simulink model "Simulation_balancenew2024versionajour"  (R2024a)
settings: Solver=ode4  StartTime=0.0  StopTime=1  FixedStep=step_time  RelTol=1e-3
InitFcn:
  | Initialisation_simulation
values from neighbouring files (symbols this model uses):
  denom_com = [R^2*C^2 3*R*C 1]    [Initialisation_simulation.m]
  denom_cou = [1/(2*pi*165) 1]    [Initialisation_simulation.m]
  denom_pos = [1/(2*pi*80) 1]    [Initialisation_simulation.m]
  denom_proc = [1,551.329784176462,25092.4669239778,5556154.83244325,117762820.943339,13657291814.2789,114001597319.831]    [Initialisation_simulation.m]
  dL_table = LUT_Table{:,6}    [Initialisation_simulation.m]
  dPhi_table = LUT_Table{:,7}    [Initialisation_simulation.m]
  gain_com = 0.88    [Initialisation_simulation.m]
  gain_cou = 0.716    [Initialisation_simulation.m]
  gain_mod_cou = Gain_Ampli_Puissance(1)    [Initialisation_simulation.m]
  gain_pos = 1.4925    [Initialisation_simulation.m]
  gain_puis = Gain_Ampli_Puissance(1)    [Initialisation_simulation.m]
  kb_table = LUT_Table{:,5}    [Initialisation_simulation.m]
  ki_courant = -325    [Initialisation_simulation.m]
  kp_courant = -0.575    [Initialisation_simulation.m]
  Lb_table = LUT_Table{:,4}    [Initialisation_simulation.m]
  num_com = 1    [Initialisation_simulation.m]
  num_cou = 1    [Initialisation_simulation.m]
  num_pos = 1    [Initialisation_simulation.m]
  num_proc = [0,0,0,-2365575.26407082,-23596424.4747652,-9504262175.32001,-113750992077.689]    [Initialisation_simulation.m]
  offset_com = -2.5    [Initialisation_simulation.m]
  offset_cou = 3.44    [Initialisation_simulation.m]
  offset_pos = -1.6    [Initialisation_simulation.m]
  per_adc = 1/freq_adc    (= 0.000166666666667)    [Initialisation_simulation.m]
  per_pwm = 1/freq_pwm    (= 6.4e-05)    [Initialisation_simulation.m]
  rb = 1.1745 + 2.349    (= 3.5235)    [Initialisation_simulation.m]
  ref_pos_act = 10    [Initialisation_simulation.m]
  ref_pos_proc = 8e-3    (= 0.008)    [Initialisation_simulation.m]
  sat_com_max = 5    [Initialisation_simulation.m]
  sat_com_min = -5    [Initialisation_simulation.m]
  sat_cou_max = 5    [Initialisation_simulation.m]
  sat_cou_min = 0    [Initialisation_simulation.m]
  sat_pos_max = 5    [Initialisation_simulation.m]
  sat_pos_min = 0    [Initialisation_simulation.m]
  sat_proc_max = 14e-3    (= 0.014)    [Initialisation_simulation.m]    (also in beam_build_ss.m = 1; lookup_table_statespace.m = 1)
  sat_proc_min = 0    [Initialisation_simulation.m]    (also in beam_build_ss.m = -1; lookup_table_statespace.m = -1)
  sat_puis_max = 5    [Initialisation_simulation.m]
  sat_puis_min = -5    [Initialisation_simulation.m]
  step_time = 1/300000    (= 3.33333333333e-06)    [Initialisation_simulation.m]
  tension_selon_distance = polyfit(Distance(1:point_final), Tension(1:point_final), 3)    [Initialisation_simulation.m]
  x_table = LUT_Table{:,2}    [Initialisation_simulation.m]
libraries: simulink_extras x2, slpidlib x2, simulink x2
settings Model: DataTypeOverride=Double  MinMaxOverflowLogging=ForceOff  Creator=johen30  LastModifiedBy=etmal6

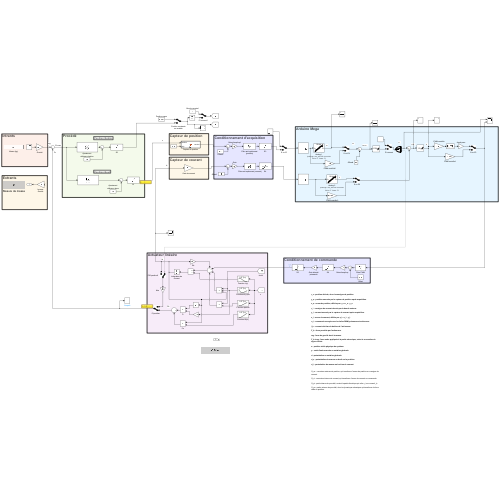
[thumbnail: Simulink's stored preview of the top-level diagram]
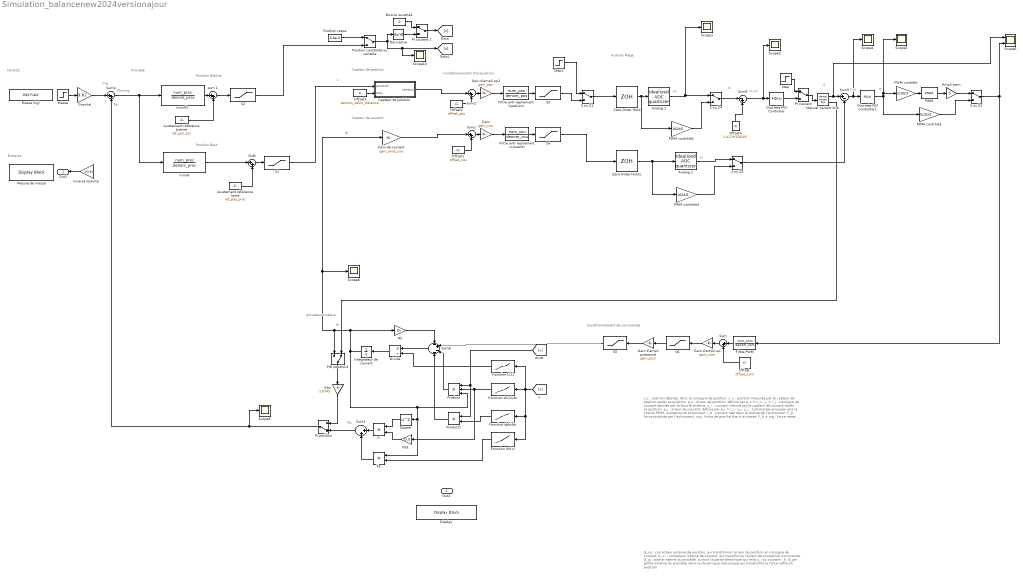
== system Simulation_balancenew2024versionajour ==
  note: G_ce : correcteur externe de position, qui transforme l’erreur de position en consigne de courant.
      |
      | G_ci : correcteur interne de courant, qui transforme l’erreur de courant en commande.
      |
      | G_pi : partie interne du procédé, surtout la partie électrique qui relie u_i au courant i_b.
      |
      | G_pe : partie externe du procédé, donc la dynamique mécanique qui transforme la force nette en position.
  note: r_x : position désirée, donc la consigne de position.
      |
      | y_x : position mesurée par le capteur de position après acquisition.
      |
      | e_x : erreur de position, définie par e_x = r_x - y_x.
      |
      | r_i : consigne de courant donnée par la boucle externe.
      |
      | y_i : courant mesuré par le capteur de courant après acquisition.
      |
      | e_i : erreur de courant, définie par e_i = r_i - y_i.
      |
      | u_i : commande envoyée vers la chaîne PWM, puissance et actionneur.
      |
      | i_b : courant réel dans la bobine de l’actionneur.
      |
      | F_b : force produite par l’actionneur.
      |
      | mg : force de gravité due à la masse.
      |
      | F_b ± mg : force nette appliquée à la partie mécanique, selon la convention de signe choisie.
      |
      | x : position réelle physique du système.
      |
      | y : sortie finale mesurée en notation générale.
      |
      | d : perturbation en notation générale.
      |
      | d_x : perturbation de mesure ou bruit sur la position.
      |
      | d_i : perturbation de mesure ou bruit sur le courant.
  note: Fb
  note: Position Bobine
  note: Extrants
  note: Intrants
  note: Arduino Mega
  note: Procédé
  note: Conditionnement de commande
  note: Conditionnement d'acquisition
  note: Actuateur linéaire
  note: Capteur de courant
  note: Capteur de position
  note: Position Bout
  note: Fb
  note: mg
  note: Fb+mg
  note: x
  note: ib
  note: ib
  note: yx
  note: yi
  note: rx
  note: ri
  note: ri-yi
  note: rx-yx
  note: ui
  Ajustement référence bobine : Constant  Value=ref_pos_act
  Ajustement référence lame : Constant  Value=ref_pos_proc
  Ampli pwm : Gain  Gain=5
  Analog 1 : simulink_extras/Additional Discrete/Idealized ADC quantizer  NumberOfConverterBits=res_adc  Vmin=0  Vmax=5  OutputDataType=int16  OutputNegativeValues=off
  Analog 2 : simulink_extras/Additional Discrete/Idealized ADC quantizer  NumberOfConverterBits=res_adc  Vmin=0  Vmax=5  OutputDataType=int16  OutputNegativeValues=off
  Boucle ouverte1 : Constant  Value=0
  Capteur de position : MATLAB Function  TreatAsAtomicUnit=on
  Derivative : Derivative
  Discrete PID Controller : slpidlib/PID Controller  Controller=PID  Form=Parallel  TimeDomain=Discrete-time  UseExternalTs=off  SampleTime=1/600  IntegratorMethod=Forward Euler  FilterMethod=Forward Euler  ControllerParametersSource=internal  P=-3.75782268839359e-06 * 200  I=-6.64373738618621e-05 * 200  UseKiTs=off  D=4.86414989946578e-07 * 200  UseExternalDerivativeSource=off  N=7.54358045778782  UseFilter=on  TunerSelectOption=Transfer Function Based (PID Tuner App)  InitialConditionSource=internal  InitialConditionForIntegrator=0  InitialConditionForFilter=0  DifferentiatorICPrevScaledInput=0  ExternalReset=none  TrackingMode=off  Kt=1  LimitOutput=on  SatLimitsSource=internal  UpperSaturationLimit=593.34  LowerSaturationLimit=0  LinearizeAsGain=off  AntiWindupMode=none  Kb=1  LimitIntegrator=off  UpperIntegratorSaturationLimit=inf  LowerIntegratorSaturationLimit=-inf  POutMin=[]  POutMax=[]  IOutMin=[]  IOutMax=[]  DOutMin=[]  DOutMax=[]  NOutMin=[]  NOutMax=[]  SumOutMin=[]  SumOutMax=[]  SaturationOutMin=[]  SaturationOutMax=[]  PParamMin=[]  PParamMax=[]  IParamMin=[]  IParamMax=[]  DParamMin=[]  DParamMax=[]  NParamMin=[]  NParamMax=[]  KbParamMin=[]  KbParamMax=[]  KtParamMin=[]  KtParamMax=[]  KbOutMin=[]  KbOutMax=[]  KtOutMin=[]  KtOutMax=[]  IntegratorOutMin=[]  IntegratorOutMax=[]  FilterOutMin=[]  FilterOutMax=[]  SumI1OutMin=[]  SumI1OutMax=[]  SumI2OutMin=[]  SumI2OutMax=[]  SumI3OutMin=[]  SumI3OutMax=[]  SumI4OutMin=[]  SumI4OutMax=[]  SumDOutMin=[]  SumDOutMax=[]  DifferentiatorOutMin=[]  DifferentiatorOutMax=[]  FilterDiffOutCoefMin=[]  FilterDiffOutCoefMax=[]  ReciprocalOutMin=[]  ReciprocalOutMax=[]  SumDenOutMin=[]  SumDenOutMax=[]  SumNumOutMin=[]  SumNumOutMax=[]  DivideOutMin=[]  DivideOutMax=[]  UdiffTsProdOutMin=[]  UdiffTsProdOutMax=[]  NTsProdOutMin=[]  NTsProdOutMax=[]  UintegralTsProdOutMin=[]  UintegralTsProdOutMax=[]  UngainTsProdOutMin=[]  UngainTsProdOutMax=[]  ClampingZeroOutDataTypeStr=Inherit: Inherit via back propagation  ClampingZeroOutMin=[]  ClampingZeroOutMax=[]  FilterDenConstantOutDataTypeStr=Inherit: Inherit via back propagation  FilterDenConstantOutMin=[]  FilterDenConstantOutMax=[]  PCopyOutDataTypeStr=Inherit: Inherit via back propagation  PCopyOutMin=[]  PCopyOutMax=[]  NCopyOutDataTypeStr=Inherit: Inherit via back propagation  NCopyOutMin=[]  NCopyOutMax=[]  IntegratorContinuousStateAttributes=''  IntegratorStateMustResolveToSignalObject=off  IntegratorRTWStateStorageClass=Auto  FilterContinuousStateAttributes=''  FilterStateMustResolveToSignalObject=off  FilterRTWStateStorageClass=Auto  ParallelPVariant=InternalParameters  IdealPVariant=Disabled  IVariant=InternalParameters  DVariant=InternalParameters  IntegratorVariant=Discrete  SatVariant=Enabled  AWVariant=Passthrough  PCopyVariant=Disabled  TRVariant=Disabled  FdbkBlocksVariant=Forward  IdealPFdbkVariant=Disabled  SatFdbkVariant=Disabled  DerivativeFilterVariant=ForwardEulerFilter  NVariant=InternalParameters  NCopyVariant=Disabled  FilterICVariant=InternalICsFilter  IntegratorICVariant=InternalICs  ExternalResetVariant=Disabled  TRSumVariant=Passthrough  SumFdbkVariant=Disabled  SumVariant=Sum_PID  TsampFilterVariant=InternalTs  TsampNgainVariant=Passthrough  TsampIntegralVariant=Disabled_SignalSpec  ExternalSaturationOutDataTypeStr=Inherit: Same as second input  DerivativeSourceVariant=ErrorSignal
      settings: LibrarySourceBlock=simulink/Discrete/Discrete PID Controller
  Discrete PID Controller1 : slpidlib/PID Controller  Controller=PI  Form=Parallel  TimeDomain=Discrete-time  UseExternalTs=off  SampleTime=1/600  IntegratorMethod=Forward Euler  FilterMethod=Forward Euler  ControllerParametersSource=internal  P=kp_courant  I=ki_courant  UseKiTs=off  D=0  UseExternalDerivativeSource=off  N=100  UseFilter=on  TunerSelectOption=Transfer Function Based (PID Tuner App)  InitialConditionSource=internal  InitialConditionForIntegrator=0  InitialConditionForFilter=0  DifferentiatorICPrevScaledInput=0  ExternalReset=none  TrackingMode=off  Kt=1  LimitOutput=on  SatLimitsSource=internal  UpperSaturationLimit=1023  LowerSaturationLimit=-1023  LinearizeAsGain=off  AntiWindupMode=none  Kb=1  LimitIntegrator=off  UpperIntegratorSaturationLimit=inf  LowerIntegratorSaturationLimit=-inf  POutMin=[]  POutMax=[]  IOutMin=[]  IOutMax=[]  DOutMin=[]  DOutMax=[]  NOutMin=[]  NOutMax=[]  SumOutMin=[]  SumOutMax=[]  SaturationOutMin=[]  SaturationOutMax=[]  PParamMin=[]  PParamMax=[]  IParamMin=[]  IParamMax=[]  DParamMin=[]  DParamMax=[]  NParamMin=[]  NParamMax=[]  KbParamMin=[]  KbParamMax=[]  KtParamMin=[]  KtParamMax=[]  KbOutMin=[]  KbOutMax=[]  KtOutMin=[]  KtOutMax=[]  IntegratorOutMin=[]  IntegratorOutMax=[]  FilterOutMin=[]  FilterOutMax=[]  SumI1OutMin=[]  SumI1OutMax=[]  SumI2OutMin=[]  SumI2OutMax=[]  SumI3OutMin=[]  SumI3OutMax=[]  SumI4OutMin=[]  SumI4OutMax=[]  SumDOutMin=[]  SumDOutMax=[]  DifferentiatorOutMin=[]  DifferentiatorOutMax=[]  FilterDiffOutCoefMin=[]  FilterDiffOutCoefMax=[]  ReciprocalOutMin=[]  ReciprocalOutMax=[]  SumDenOutMin=[]  SumDenOutMax=[]  SumNumOutMin=[]  SumNumOutMax=[]  DivideOutMin=[]  DivideOutMax=[]  UdiffTsProdOutMin=[]  UdiffTsProdOutMax=[]  NTsProdOutMin=[]  NTsProdOutMax=[]  UintegralTsProdOutMin=[]  UintegralTsProdOutMax=[]  UngainTsProdOutMin=[]  UngainTsProdOutMax=[]  ClampingZeroOutDataTypeStr=Inherit: Inherit via back propagation  ClampingZeroOutMin=[]  ClampingZeroOutMax=[]  FilterDenConstantOutDataTypeStr=Inherit: Inherit via back propagation  FilterDenConstantOutMin=[]  FilterDenConstantOutMax=[]  PCopyOutDataTypeStr=Inherit: Inherit via back propagation  PCopyOutMin=[]  PCopyOutMax=[]  NCopyOutDataTypeStr=Inherit: Inherit via back propagation  NCopyOutMin=[]  NCopyOutMax=[]  IntegratorContinuousStateAttributes=''  IntegratorStateMustResolveToSignalObject=off  IntegratorRTWStateStorageClass=Auto  FilterContinuousStateAttributes=''  FilterStateMustResolveToSignalObject=off  FilterRTWStateStorageClass=Auto  ParallelPVariant=InternalParameters  IdealPVariant=Disabled  IVariant=InternalParameters  DVariant=Disabled  IntegratorVariant=Discrete  SatVariant=Enabled  AWVariant=Passthrough  PCopyVariant=Disabled  TRVariant=Disabled  FdbkBlocksVariant=Forward  IdealPFdbkVariant=Disabled  SatFdbkVariant=Disabled  DerivativeFilterVariant=Disabled  NVariant=Disabled  NCopyVariant=Disabled_SignalSpec  FilterICVariant=Disabled  IntegratorICVariant=InternalICs  ExternalResetVariant=Disabled  TRSumVariant=Passthrough  SumFdbkVariant=Disabled  SumVariant=Sum_PI  TsampFilterVariant=InternalTs  TsampNgainVariant=Passthrough  TsampIntegralVariant=Disabled_SignalSpec  ExternalSaturationOutDataTypeStr=Inherit: Same as second input  DerivativeSourceVariant=Disabled
      settings: LibrarySourceBlock=simulink/Discrete/Discrete PID Controller
  Display : DisplayBlock  LabelPosition=Hide  Transparency=1
  Divide : Product  Inputs=*/
  Fa : Product
  Fi : Product
  Filtre PWM : TransferFcn  Numerator=num_com  Denominator=denom_com
  Filtre anti-repliement (position) : TransferFcn  Numerator=num_pos  Denominator=denom_pos
  Filtre anti-repliement (courant) : TransferFcn  Numerator=num_cou  Denominator=denom_cou
  Fonction Kb(x) : Lookup_n-D  NumberOfTableDimensions=1  BreakpointsForDimension1=x_table  Table=kb_table  InternalRulePriority=Speed  RndMeth=Simplest
  Fonction L(x) : Lookup_n-D  NumberOfTableDimensions=1  BreakpointsForDimension1=x_table  Table=Lb_table  InternalRulePriority=Speed  RndMeth=Simplest
  Fonction dL(x)/dx : Lookup_n-D  NumberOfTableDimensions=1  BreakpointsForDimension1=x_table  Table=dL_table  InternalRulePriority=Speed  RndMeth=Simplest
  Fonction dphi/dx : Lookup_n-D  NumberOfTableDimensions=1  BreakpointsForDimension1=x_table  Table=dPhi_table  InternalRulePriority=Speed  RndMeth=Simplest
  Gain : Gain  Gain=gain_cou
  Gain d'ampli puissance : Gain  Gain=gain_puis
  Gain d'ampli-op : Gain  Gain=gain_com
  Gain d'ampli-op1 : Gain  Gain=gain_pos
  Gain de courant : Gain  Gain=gain_mod_cou
  Gravité : Gain  Gain=9.81
  Intégrateur de courant : Integrator
  Inverse Gravité : Gain  Gain=1/9.81
  Kbo : Gain  Gain=-1.0745
  Manual Variant Sink : simulink/Signal Routing/Manual Variant Sink  NumChoices=2  LabelModeActiveChoice=V_1
  Masse : Step  After=0.05  SampleTime=0
  Masse (kg) : EditField  LabelPosition=Hide  ShowInitialText=on  Alignment=Center
  Mesure de masse : DisplayBlock  LabelPosition=Hide  Transparency=1
  Offset : Constant  Value=offset_com
  Offset1 : Constant  Value=offset_cou
  Offset2 : Constant  Value=offset_pos
  Offset3 : Constant  Value=tension_selon_distance
  Offset4 : Constant  Value=1.4174*1023/5
  PI courant : ManualSwitch
  PI courant 1 : ManualSwitch
  PI position : ManualSwitch  CurrentSetting=0
  "PID position2 " : ManualSwitch  CurrentSetting=0
  PWM : simulink/Discontinuities/PWM  DisableCoverage=on  Period=per_pwm  InitialDelay=0  DisallowZeroDutyCycle=off  RunAtFixedTimeIntervals=on  SampleTime=step_time
  PWM contrôle : Gain  Gain=1/1023  OutDataTypeStr=fixdt(1,64, 44)
  PWM contrôle1 : Gain  Gain=5/1023  OutDataTypeStr=fixdt(1,64, 44)
  PWM contrôle2 : Gain  Gain=1023/5  OutDataTypeStr=fixdt(1,64, 44)
  PWM contrôle3 : Gain  Gain=1023/5  OutDataTypeStr=fixdt(1,64, 44)
  Position constante ou variable : ManualSwitch
  Position repos : Constant  Value=6.6e-3
  Product : Product  Inputs=3
  Product1 : Product
  Rb : Gain  Gain=rb
  Rb1 : Gain  Gain=0.5
  S ou Z{1,3..5} (4 alike) : ManualSwitch
  S1 : Saturate  UpperLimit=sat_proc_max  LowerLimit=sat_proc_min  LinearizeAsGain=off
  S2 : Saturate  UpperLimit=sat_proc_max  LowerLimit=sat_proc_min  LinearizeAsGain=off
  S3 : Saturate  UpperLimit=sat_pos_max  LowerLimit=sat_pos_min  LinearizeAsGain=off
  S4 : Saturate  UpperLimit=sat_cou_max  LowerLimit=sat_cou_min
  S5 : Saturate  UpperLimit=sat_puis_max  LowerLimit=sat_puis_min
  S6 : Saturate  UpperLimit=sat_com_max  LowerLimit=sat_com_min
  SUM : Sum  Inputs=|++
  Scope{1..2,4..5,8..10} (7 alike) : Scope
  Scope6 : Scope  NumInputPorts=2
  Square : Math  Operator=square
  Step : Step  Time=0.01  After=5  SampleTime=0
  Step1 : Step  After=2  SampleTime=0
  Sum{,1..4} (5 alike) : Sum  Inputs=|++
  Sum5 : Sum  Inputs=|+-
  Sum6 : Sum  Inputs=-+--
  Sum8 : Sum  Inputs=|-+
  Zero-Order Hold : ZeroOrderHold  SampleTime=per_adc
  Zero-Order Hold1 : ZeroOrderHold  SampleTime=per_adc
  mm/N : TransferFcn  Numerator=num_proc  Denominator=denom_proc
  mm/N1 : TransferFcn  Numerator=num_proc  Denominator=denom_proc
  sum 1 : Sum  Inputs=|++
  Out1 : Outport
  Out2 : Outport  Port=2
  wires:
  Offset1/1 -> Sum1/2
  Gain d'ampli-op1/1 -> Filtre anti-repliement (position)/1
  Filtre anti-repliement (position)/1 -> S3/1
  Sum2/1 -> Gain d'ampli-op1/1
  Sum1/1 -> Gain/1
  Gain d'ampli puissance/1 -> S5/1
  Sum4/1 -> mm/N1/1, mm/N/1
  Zero-Order Hold/1 -> PWM contrôle2/1, Analog 1/1
  Zero-Order Hold1/1 -> PWM contrôle3/1, Analog 2/1
  PWM/1 -> Ampli pwm/1
  Offset/1 -> Sum/2
  S6/1 -> Gain d'ampli puissance/1
  Divide/1 -> Intégrateur de courant/1
  Sum6/1 -> Divide/1
  Rb/1 -> Sum6/1
  [x] -> Fonction dL(x)/dx/1, Fonction L(x)/1, Fonction dphi/dx/1, Fonction Kb(x)/1
  Fonction L(x)/1 -> Divide/2
  [v] -> Product/1, Product1/1
  Fonction dL(x)/dx/1 -> Rb1/1, Product/2
  Fonction dphi/dx/1 -> Product1/2
  Product1/1 -> Sum6/4
  Product/1 -> Sum6/3
  Offset2/1 -> Sum2/2
  Gain/1 -> Filtre anti-repliement (courant)/1
  Filtre anti-repliement (courant)/1 -> S4/1
  PWM contrôle/1 -> PWM/1
  Filtre PWM/1 -> Sum/1
  Gain d'ampli-op/1 -> S6/1
  Sum/1 -> Gain d'ampli-op/1
  Offset3/1 -> Capteur de position/2(poly)
  Intégrateur de courant/1 -> Rb/1, Scope8/1, Gain de courant/1, "PID position2 "/1, Fa/1, Square/1, Product/3
  mm/N1/1 -> sum 1/1
  sum 1/1 -> S2/1
  Ajustement référence lame/1 -> SUM/2
  Ajustement référence bobine/1 -> sum 1/2
  Gain de courant/1 -> Sum1/1
  Inverse Gravité/1 -> Out1/1
  Square/1 -> Fi/1
  Rb1/1 -> Fi/2
  Fonction Kb(x)/1 -> Fa/2
  Fi/1 -> Sum3/1
  Fa/1 -> Sum3/2
  Position constante ou variable/1 -> Derivative/1, Scope10/1, [x]
  Position repos/1 -> Position constante ou variable/1
  S ou Z3/1 -> Scope6/2, Filtre PWM/1
  Masse/1 -> Gravité/1
  S4/1 -> Zero-Order Hold1/1
  Gravité/1 -> Sum4/1
  SUM/1 -> S1/1
  mm/N/1 -> SUM/1
  Capteur de position/1(tension) -> Sum2/1
  Offset4/1 -> Sum8/2
  Analog 1/1 -> S ou Z4/1, Scope1/1
  Discrete PID Controller1/1 -> PWM contrôle/1, Scope5/1, PWM contrôle1/1
  Boucle ouverte1/1 -> PI courant 1/1
  Derivative/1 -> PI courant 1/2
  PI courant 1/1 -> [v]
  Discrete PID Controller/1 -> PI courant/2
  Step/1 -> PI courant/1
  Ampli pwm/1 -> S ou Z3/1
  PWM contrôle1/1 -> S ou Z3/2
  Sum5/1 -> Scope4/1, Discrete PID Controller1/1
  Analog 2/1 -> S ou Z5/1
  S ou Z5/1 -> Sum5/2
  PWM contrôle3/1 -> S ou Z5/2
  Sum8/1 -> Scope2/1, Discrete PID Controller/1
  PWM contrôle2/1 -> S ou Z4/2
  S ou Z4/1 -> Sum8/1
  Sum3/1 -> PI position/2
  PI position/1 -> Scope9/1, Sum4/2
  Kbo/1 -> PI position/1
  S2/1 -> Position constante ou variable/2
  S1/1 -> Capteur de position/1(position)
  "PID position2 "/1 -> Kbo/1
  PI courant/1 -> Manual Variant Sink/1
  Manual Variant Sink/1 -> Scope6/1, Sum5/1
  Manual Variant Sink/2 -> "PID position2 "/2
  S5/1 -> Sum6/2
  S ou Z1/1 -> Zero-Order Hold/1
  S3/1 -> S ou Z1/2
  Step1/1 -> S ou Z1/1

== matlab function Simulation_balancenew2024versionajour/Capteur de position ==
  data: position input; tension output; poly input
function tension = fct(position, poly)

tension = polyval(poly, position);
